simulink model "QuadSimControl"  (R2025a)
settings: Solver=VariableStepAuto  StartTime=0.0  StopTime=700  RelTol=1e-3
undefined symbols (not defined in the file): Ts_c
libraries: SignalEditorBlockLib x3, simulink_extras x2, sharedtransform x1, uavutilslib x1
settings Model: Creator=User  LastModifiedBy=luke

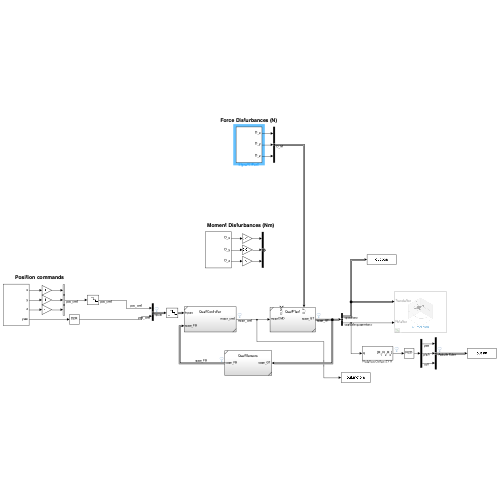
[thumbnail: Simulink's stored preview of the top-level diagram]
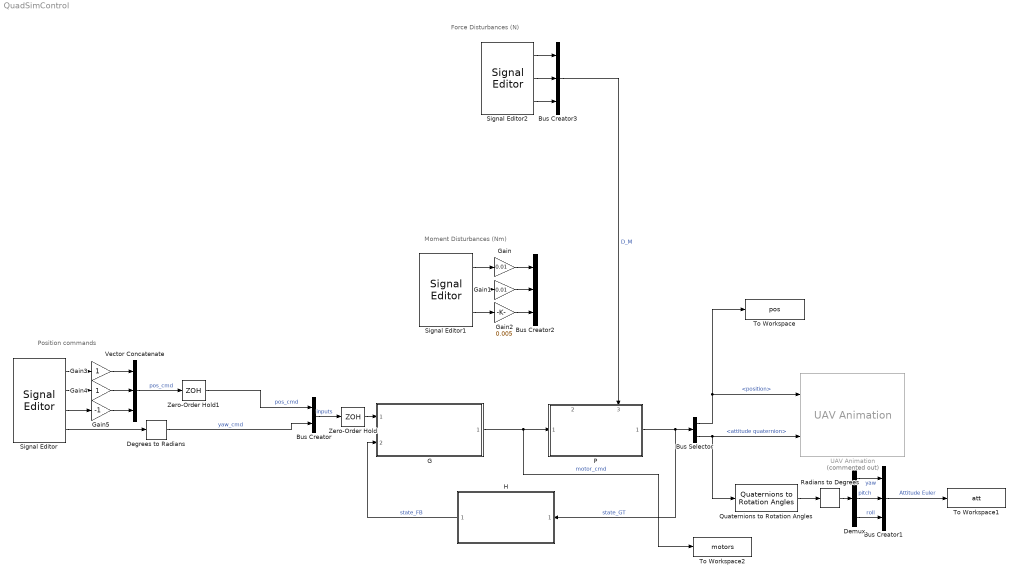
== system QuadSimControl ==
  note: Position commands
  note: Moment Disturbances (Nm)
  note: Force Disturbances (N)
  Bus Creator : BusCreator  Inputs=2
  Bus Creator1 : BusCreator  Inputs=3
  Bus Creator2 : BusCreator  Inputs=3
  Bus Creator3 : BusCreator  Inputs=3
  Bus Selector : BusSelector  OutputSignals=Translation State.position,Attitude State.attitude quaternion
  Degrees to Radians : simulink_extras/Transformations/Degrees to Radians
  Demux : Demux  Outputs=3
  G : Subsystem  ReferencedSubsystem=QuadController
  Gain : Gain  Gain=0.01
  Gain1 : Gain  Gain=0.01
  Gain2 : Gain  Gain=0.005
  Gain3 : Gain
  Gain4 : Gain
  Gain5 : Gain  Gain=-1
  H : Subsystem  ReferencedSubsystem=QuadSensors
  P : Subsystem  ReferencedSubsystem=QuadPlant
      settings: PortSchema="{\"entries\":[{\"content\":{\"sides\":[{\"content\":{\"connectorIds\":[\"In1\"]},\"type\":\"ConnectorPlacement.EquallySpacedRectSide\",\"uuid\":\"75791568-d9a2-45b2-910f-6e38cddb082e\"},{\"content\":{\"connectorIds\":[\"Out1\"],\"side\":\"RIGHT\"},\"type\":\"ConnectorPlacement.EquallySpacedRectSide\",\"uuid\":\"1a224a0c-a8d6-4b18-8919-171d6140d7a5\"},{\"content\":{\"connectorIds\":[\"In2\",\"In3\"],\"side\":\"TOP\"},\"type\":\"ConnectorPlacement.EquallySpacedRectSide\",\"uuid\":\"5f468aca-e0c4-4a85-891e-cda82e48e898\"}]},\"type\":\"ConnectorPlacement.EquallySpacedConnector\",\"uuid\":\"30894ac3-ed23-4729-ac12-eeea0dfad17c\"}],\"packageUris\":[\"http://schema.mathworks.com/mf0/Connector/R2020b\"],\"version\":\"1.0\"}"
  Quaternions to Rotation Angles : sharedtransform/Quaternions to Rotation Angles  rotationOrder=ZYX  aMode=aMode
  Radians to Degrees : simulink_extras/Transformations/Radians to Degrees
  Signal Editor : SignalEditorBlockLib/Signal Editor  FileName=ShortReferenceSteps.mat  ActiveScenario=Scenario  ActiveSignal=x  IsBus=off  OutputBusObjectStr=Bus: BusObject  SampleTime=0  ZeroCross=off  OutputAfterFinalValue=Setting to zero  Unit=inherit  PreserveSignalName=on  ApplySigPropsToAllScenarios=on  ApplySigPropsToAllSignals=off  SignalPropertySource=Dialog parameters
  Signal Editor1 : SignalEditorBlockLib/Signal Editor  FileName=MomentDisturbanceSteps.mat  ActiveScenario=Scenario  ActiveSignal=D_x  IsBus=off  OutputBusObjectStr=Bus: BusObject  SampleTime=0  ZeroCross=off  OutputAfterFinalValue=Setting to zero  Unit=inherit  PreserveSignalName=on  ApplySigPropsToAllScenarios=on  ApplySigPropsToAllSignals=off  SignalPropertySource=Dialog parameters
  Signal Editor2 : SignalEditorBlockLib/Signal Editor  FileName=MomentDisturbanceSteps.mat  ActiveScenario=Scenario  ActiveSignal=D_x  IsBus=off  OutputBusObjectStr=Bus: BusObject  SampleTime=0  ZeroCross=off  OutputAfterFinalValue=Setting to zero  Unit=inherit  PreserveSignalName=on  ApplySigPropsToAllScenarios=on  ApplySigPropsToAllSignals=off  SignalPropertySource=Dialog parameters
  To Workspace : ToWorkspace  VariableName=pos  SaveFormat=Structure With Time  SampleTime=0.01
  To Workspace1 : ToWorkspace  VariableName=att  SaveFormat=Structure With Time  SampleTime=0.01
  To Workspace2 : ToWorkspace  VariableName=motors  SaveFormat=Structure With Time  SampleTime=0.005
  UAV Animation : uavutilslib/UAV Animation  Commented=on  NumUAV=1  DynamicUAVConfig=off  UAVType=Multirotor  UAVSize=1  UAVColor=[1 0 0]  UAVTrajectoryAlpha=1  InertialZDirection=Down  RotationFormat=Quaternion  DrawMarkers=off  SampleTime=0.05
  Vector Concatenate : Concatenate  NumInputs=3
  Zero-Order Hold : ZeroOrderHold  SampleTime=Ts_c
  Zero-Order Hold1 : ZeroOrderHold  SampleTime=Ts_c
  wires:
  P/1 -> H/1, Bus Selector/1  "state_GT"
  Bus Creator/1 -> Zero-Order Hold/1  "inputs"
  G/1 -> To Workspace2/1, P/1  "motor_cmd"
  Bus Selector/2 -> UAV Animation/2, Quaternions to Rotation Angles/1  "<attitude quaternion>"
  Degrees to Radians/1 -> Bus Creator/2  "yaw_cmd"
  Quaternions to Rotation Angles/1 -> Radians to Degrees/1
  H/1 -> G/2  "state_FB"
  Demux/1 -> Bus Creator1/1  "yaw"
  Demux/2 -> Bus Creator1/2  "pitch"
  Demux/3 -> Bus Creator1/3  "roll"
  Bus Creator1/1 -> To Workspace1/1  "Attitude Euler"
  Radians to Degrees/1 -> Demux/1
  Zero-Order Hold/1 -> G/1
  Vector Concatenate/1 -> Zero-Order Hold1/1  "pos_cmd"
  Bus Selector/1 -> To Workspace/1, UAV Animation/1  "<position>"
  Zero-Order Hold1/1 -> Bus Creator/1  "pos_cmd"
  Signal Editor/4 -> Degrees to Radians/1
  Signal Editor2/1 -> Bus Creator3/1
  Signal Editor2/2 -> Bus Creator3/2
  Signal Editor2/3 -> Bus Creator3/3
  Signal Editor1/1 -> Gain/1
  Signal Editor1/2 -> Gain1/1
  Signal Editor1/3 -> Gain2/1
  Gain/1 -> Bus Creator2/1
  Gain1/1 -> Bus Creator2/2
  Gain2/1 -> Bus Creator2/3
  Signal Editor/1 -> Gain3/1
  Signal Editor/2 -> Gain4/1
  Gain3/1 -> Vector Concatenate/1
  Gain4/1 -> Vector Concatenate/2
  Signal Editor/3 -> Gain5/1
  Gain5/1 -> Vector Concatenate/3
  Bus Creator3/1 -> P/3  "D_M"
